simulink model "quarter_suspension"  (R2020b)
settings: Solver=VariableStepAuto  StartTime=0.0  StopTime=10.0  RelTol=1e-3
settings Model: Creator=sharad  LastModifiedBy=anishabhangui
settings DataIOCC: ReturnWorkspaceOutputs=off
settings DebuggingCC: ArithmeticOperatorsInVariantConditions=warning
settings SFSimCC: SimUseLocalCustomCode=off  CustomCodeUndefinedFunction=UseInterfaceOnly
settings RTWCC: RTWUseLocalCustomCode=off

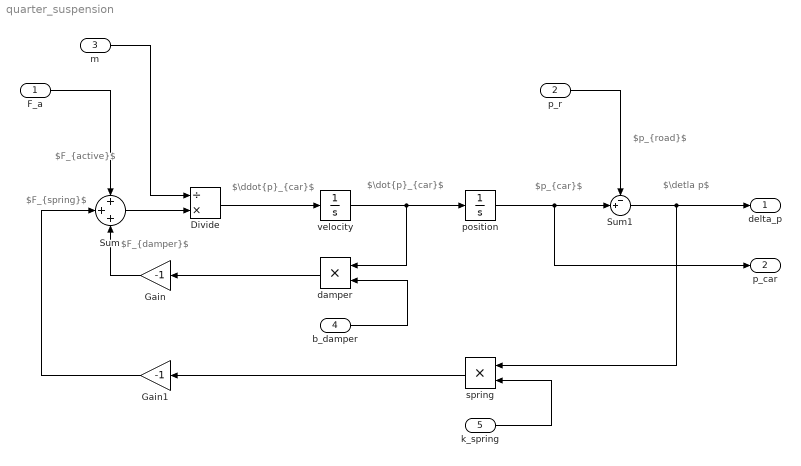
== system quarter_suspension ==
  note: $F_{spring}$
  note: $F_{damper}$
  note: $F_{active}$
  note: $p_{road}$
  note: $p_{car}$
  note: $\detla p$
  note: $\dot{p}_{car}$
  note: $\ddot{p}_{car}$
  F_a : Inport
  p_r : Inport  Port=2
  m : Inport  Port=3
  b_damper : Inport  Port=4
  k_spring : Inport  Port=5
  Divide : Product  Inputs=/*
  Gain : Gain  Gain=-1
  Gain1 : Gain  Gain=-1
  Sum : Sum  Inputs=+++
  Sum1 : Sum  Inputs=-+|
  damper : Product
  position : Integrator
  spring : Product
  velocity : Integrator
  delta_p : Outport  VectorParamsAs1DForOutWhenUnconnected=off
  p_car : Outport  Port=2  VectorParamsAs1DForOutWhenUnconnected=off
  wires:
  velocity/1 -> damper/1, position/1
  position/1 -> p_car/1, Sum1/2
  p_r/1 -> Sum1/1
  damper/1 -> Gain/1
  b_damper/1 -> damper/2
  spring/1 -> Gain1/1
  k_spring/1 -> spring/2
  Sum1/1 -> spring/1, delta_p/1
  Gain1/1 -> Sum/2
  Sum/1 -> Divide/2
  Divide/1 -> velocity/1
  m/1 -> Divide/1
  Gain/1 -> Sum/3
  F_a/1 -> Sum/1
